simulink model "Simulink_Group23_Fuzzy"  (R2021a)
settings: Solver=FixedStepAuto  StartTime=0.0  StopTime=10.0  FixedStep=0.01  RelTol=1e-3
libraries: fuzblock x1
settings Model: Creator=asus  LastModifiedBy=asus

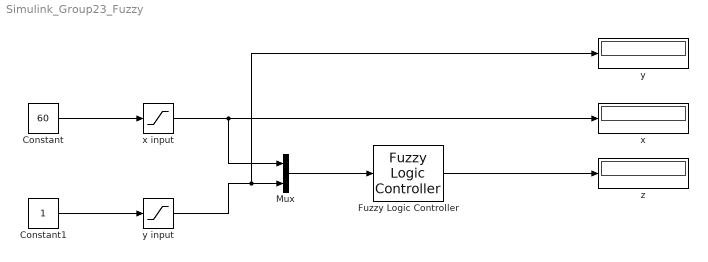
== system Simulink_Group23_Fuzzy ==
  Constant : Constant  Value=60
  Constant1 : Constant
  Fuzzy Logic Controller : fuzblock/Fuzzy Logic  Controller  FIS='Group23_Fuzzy.fis'  OutputSampleNumber=101  DataType=double  FuzzifiedInputs=off  RuleFiringStrengths=off  RuleOutputs=off  AggregatedOutputs=off  SimulateUsing=Interpreted execution  OutOfRangeInputValueMessage=warning  NoRuleFiredMessage=warning  EmptyOutputFuzzySetMessage=warning
  Mux : Mux  Inputs=2
  x : Display
  x input : Saturate  UpperLimit=60  LowerLimit=0
  y : Display
  y input : Saturate  UpperLimit=3  LowerLimit=0
  z : Display
  wires:
  Mux/1 -> Fuzzy Logic Controller/1
  y input/1 -> y/1, Mux/2
  x input/1 -> Mux/1, x/1
  Constant/1 -> x input/1
  Constant1/1 -> y input/1
  Fuzzy Logic Controller/1 -> z/1
